simulink model "lab01"  (R2021a)
settings: Solver=VariableStepAuto  StartTime=0.0  StopTime=10  RelTol=1e-3
model workspace (MAT data in the model file):
  T0 = 0.4
values from neighbouring files (symbols this model uses):
  g = 9.8    [lab02.mat]    (also in lab03.mat; lab04.mat; lab05.mat; lab06.mat)
  Ja = 0.06904489    [lab02.mat]    (also in lab03.mat; lab04.mat; lab05.mat = 0.06191089; lab06.mat = 0.06932089)
  Jb = 0.04317025    [lab02.mat]    (also in lab03.mat; lab04.mat; lab05.mat = 0.03603625; lab06.mat = 0.04344625)
  l_0 = 0.33    [lab02.mat]    (also in lab03.mat; lab04.mat; lab05.mat; lab06.mat)
  l_c = -0.0458067226891    [lab03.mat]    (also in lab04.mat; lab05.mat = -0.0295602240896; lab06.mat = -0.0463669467787; lab07.mat = -0.0295602240896)
  m_1 = 0.2376    [lab02.mat]    (also in lab03.mat; lab04.mat; lab05.mat; lab06.mat)
  m_2 = 1.785    [lab02.mat]    (also in lab03.mat; lab04.mat; lab05.mat; lab06.mat)
undefined symbols (not defined in the file or in its folder): Den, F, Num, T_0
settings Model: Creator=kisdev  LastModifiedBy=kisdev

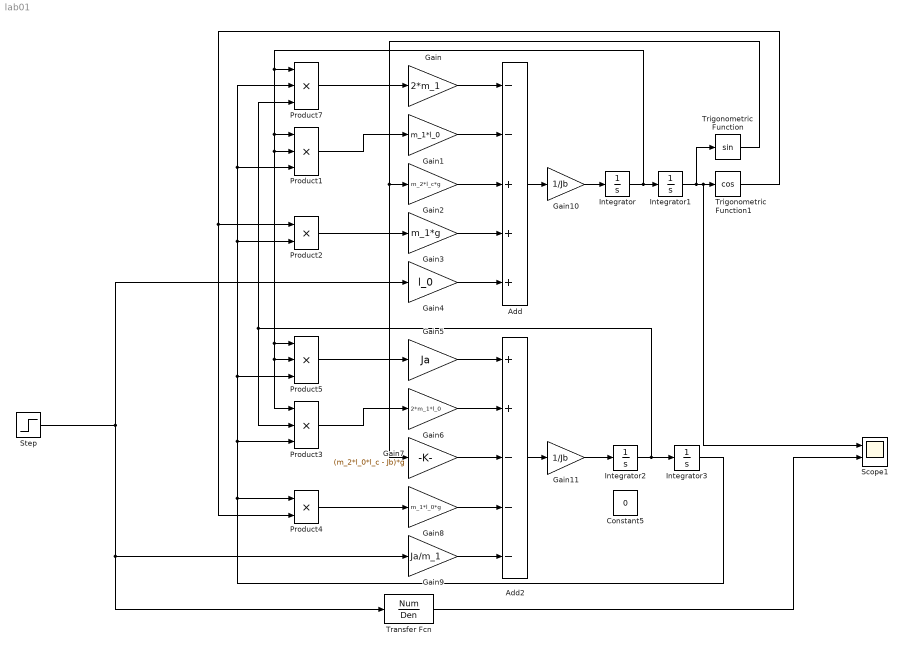
== system lab01 ==
  Add : Sum  Inputs=--+++
  Add2 : Sum  Inputs=++---
  Constant5 : Constant  Value=0
  Gain : Gain  Gain=2*m_1
  Gain1 : Gain  Gain=m_1*l_0
  Gain10 : Gain  Gain=1/Jb
  Gain11 : Gain  Gain=1/Jb
  Gain2 : Gain  Gain=m_2*l_c*g
  Gain3 : Gain  Gain=m_1*g
  Gain4 : Gain  Gain=l_0
  Gain5 : Gain  Gain=Ja
  Gain6 : Gain  Gain=2*m_1*l_0
  Gain7 : Gain  Gain=(m_2*l_0*l_c - Jb)*g
  Gain8 : Gain  Gain=m_1*l_0*g
  Gain9 : Gain  Gain=Ja/m_1
  Integrator : Integrator
  Integrator1 : Integrator  InitialCondition=T_0
  Integrator2 : Integrator
  Integrator3 : Integrator
  Product{1,3,5,7} (4 alike) : Product  Inputs=3
  Product2 : Product
  Product4 : Product
  Scope1 : Scope  NumInputPorts=2
  Step : Step  Time=0  After=F  SampleTime=0
  Transfer Fcn : TransferFcn  Numerator=Num  Denominator=Den
  Trigonometric Function : Trigonometry
  Trigonometric Function1 : Trigonometry  Operator=cos
  wires:
  Integrator2/1 -> Integrator3/1, Product3/2, Product7/3
  Integrator/1 -> Product1/1, Product3/1, Product5/2, Product5/1, Product1/2, Product7/1, Integrator1/1
  Integrator1/1 -> Scope1/1, Trigonometric Function1/1, Trigonometric Function/1
  Gain/1 -> Add/1
  Gain1/1 -> Add/2
  Gain2/1 -> Add/3
  Gain3/1 -> Add/4
  Gain4/1 -> Add/5
  Gain5/1 -> Add2/1
  Gain6/1 -> Add2/2
  Gain7/1 -> Add2/3
  Gain8/1 -> Add2/4
  Gain9/1 -> Add2/5
  Integrator3/1 -> Product4/1, Product3/3, Product5/3, Product2/2, Product1/3, Product7/2
  Product7/1 -> Gain/1
  Product1/1 -> Gain1/1
  Trigonometric Function/1 -> Gain7/1, Gain2/1
  Product2/1 -> Gain3/1
  Trigonometric Function1/1 -> Product2/1, Product4/2
  Step/1 -> Transfer Fcn/1, Gain9/1, Gain4/1
  Product5/1 -> Gain5/1
  Product3/1 -> Gain6/1
  Product4/1 -> Gain8/1
  Add/1 -> Gain10/1
  Gain10/1 -> Integrator/1
  Add2/1 -> Gain11/1
  Gain11/1 -> Integrator2/1
  Transfer Fcn/1 -> Scope1/2
